simulink model "test_other_torques_sim"  (R2021b)
settings: Solver=ode8  StartTime=0.0  StopTime=1000  FixedStep=0.01  RelTol=1e-3
values from neighbouring files (symbols this model uses):
  alfaG = 0    [test_other_torques_var.m]
  m = [0.1 0.1 0.1]'    [test_other_torques_var.m]
libraries: environment x5, orbit x3, kinematics x3, dynamics x3, my_math_ops x2
settings Model: Creator=Davide  LastModifiedBy=Davide

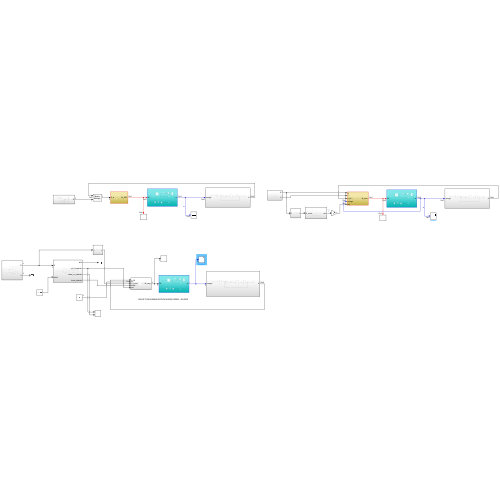
[thumbnail: Simulink's stored preview of the top-level diagram]
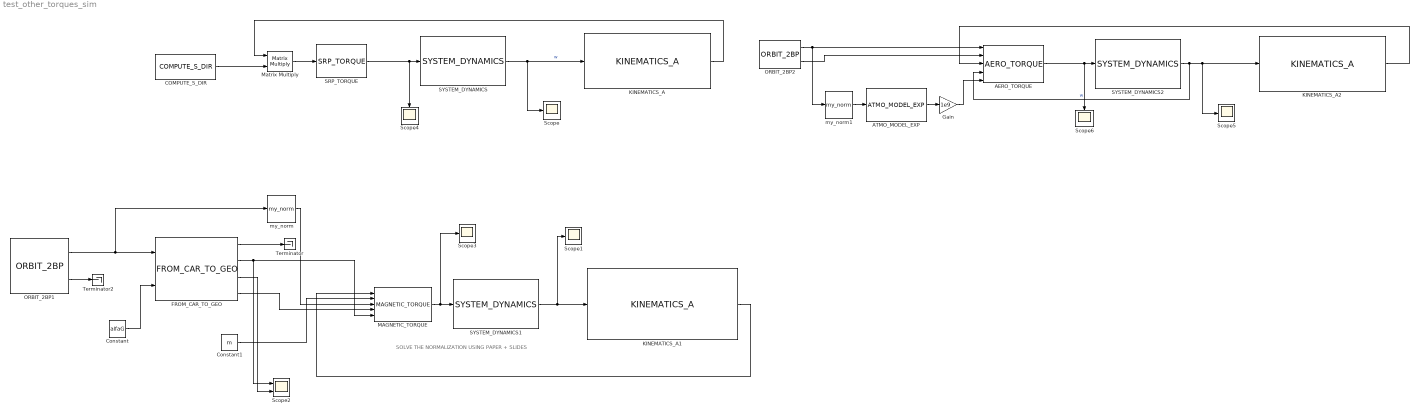
== system test_other_torques_sim ==
  note: SOLVE THE NORMALIZATION USING PAPER + SLIDES
  AERO_TORQUE : environment/AERO_TORQUE  SystemSampleTime=-1  VariantActivationTime=update diagram  Latency=0  AutoFrameSizeCalculation=off
      settings: SourceProductName=Environment
  ATMO_MODEL_EXP : environment/ATMO_MODEL_EXP  SystemSampleTime=-1  VariantActivationTime=update diagram  Latency=0  AutoFrameSizeCalculation=off
      settings: SourceProductName=Environment
  COMPUTE_S_DIR : environment/COMPUTE_S_DIR  SystemSampleTime=-1  VariantActivationTime=update diagram  Latency=0  AutoFrameSizeCalculation=off
      settings: SourceProductName=Environment
  Constant : Constant  Value=alfaG
  Constant1 : Constant  Value=m
  FROM_CAR_TO_GEO : orbit/FROM_CAR_TO_GEO  SystemSampleTime=-1  VariantActivationTime=update diagram  Latency=0  AutoFrameSizeCalculation=off
      settings: SourceProductName=Orbit
  Gain : Gain  Gain=1e9
  KINEMATICS_A : kinematics/KINEMATICS_A  SystemSampleTime=-1  VariantActivationTime=update diagram  Latency=0  AutoFrameSizeCalculation=off
      settings: SourceProductName=Kinematics
  KINEMATICS_A1 : kinematics/KINEMATICS_A  SystemSampleTime=-1  VariantActivationTime=update diagram  Latency=0  AutoFrameSizeCalculation=off
      settings: SourceProductName=Kinematics
  KINEMATICS_A2 : kinematics/KINEMATICS_A  SystemSampleTime=-1  VariantActivationTime=update diagram  Latency=0  AutoFrameSizeCalculation=off
      settings: SourceProductName=Kinematics
  MAGNETIC_TORQUE : environment/MAGNETIC_TORQUE  SystemSampleTime=-1  VariantActivationTime=update diagram  Latency=0  AutoFrameSizeCalculation=off
      settings: SourceProductName=Environment
  Matrix Multiply : Product  Multiplication=Matrix(*)
  ORBIT_2BP1 : orbit/ORBIT_2BP  SystemSampleTime=-1  VariantActivationTime=update diagram  Latency=0  AutoFrameSizeCalculation=off
      settings: SourceProductName=Orbit
  ORBIT_2BP2 : orbit/ORBIT_2BP  SystemSampleTime=-1  VariantActivationTime=update diagram  Latency=0  AutoFrameSizeCalculation=off
      settings: SourceProductName=Orbit
  SRP_TORQUE : environment/SRP_TORQUE  SystemSampleTime=-1  VariantActivationTime=update diagram  Latency=0  AutoFrameSizeCalculation=off
      settings: SourceProductName=Environment
  SYSTEM_DYNAMICS : dynamics/SYSTEM_DYNAMICS  SystemSampleTime=-1  VariantActivationTime=update diagram  Latency=0  AutoFrameSizeCalculation=off
      settings: SourceProductName=Dynamics
  SYSTEM_DYNAMICS1 : dynamics/SYSTEM_DYNAMICS  SystemSampleTime=-1  VariantActivationTime=update diagram  Latency=0  AutoFrameSizeCalculation=off
      settings: SourceProductName=Dynamics
  SYSTEM_DYNAMICS2 : dynamics/SYSTEM_DYNAMICS  SystemSampleTime=-1  VariantActivationTime=update diagram  Latency=0  AutoFrameSizeCalculation=off
      settings: SourceProductName=Dynamics
  Scope{,1,3..6} (6 alike) : Scope
  Scope2 : Scope  NumInputPorts=2
  Terminator : Terminator
  Terminator2 : Terminator
  my_norm : my_math_ops/my_norm  SystemSampleTime=-1  VariantActivationTime=update diagram  Latency=0  AutoFrameSizeCalculation=off
      settings: SourceProductName=My Mathematics Operations
  my_norm1 : my_math_ops/my_norm  SystemSampleTime=-1  VariantActivationTime=update diagram  Latency=0  AutoFrameSizeCalculation=off
      settings: SourceProductName=My Mathematics Operations
  wires:
  SRP_TORQUE/1 -> Scope4/1, SYSTEM_DYNAMICS/1
  SYSTEM_DYNAMICS/1 -> Scope/1, KINEMATICS_A/1  "w"
  KINEMATICS_A1/1 -> MAGNETIC_TORQUE/1
  SYSTEM_DYNAMICS1/1 -> Scope1/1, KINEMATICS_A1/1
  MAGNETIC_TORQUE/1 -> Scope3/1, SYSTEM_DYNAMICS1/1
  ORBIT_2BP1/1 -> my_norm/1, FROM_CAR_TO_GEO/1
  FROM_CAR_TO_GEO/3 -> Scope2/2
  FROM_CAR_TO_GEO/2 -> Scope2/1, MAGNETIC_TORQUE/5
  FROM_CAR_TO_GEO/1 -> Terminator/1
  FROM_CAR_TO_GEO/4 -> MAGNETIC_TORQUE/4
  Constant/1 -> FROM_CAR_TO_GEO/2
  ORBIT_2BP1/2 -> Terminator2/1
  Constant1/1 -> MAGNETIC_TORQUE/2
  my_norm/1 -> MAGNETIC_TORQUE/3
  COMPUTE_S_DIR/1 -> Matrix Multiply/2
  KINEMATICS_A/1 -> Matrix Multiply/1
  Matrix Multiply/1 -> SRP_TORQUE/1
  ORBIT_2BP2/1 -> AERO_TORQUE/1, my_norm1/1
  ORBIT_2BP2/2 -> AERO_TORQUE/2
  KINEMATICS_A2/1 -> AERO_TORQUE/3
  AERO_TORQUE/1 -> Scope6/1, SYSTEM_DYNAMICS2/1
  SYSTEM_DYNAMICS2/1 -> AERO_TORQUE/4, Scope5/1, KINEMATICS_A2/1  "w"
  my_norm1/1 -> ATMO_MODEL_EXP/1
  ATMO_MODEL_EXP/1 -> Gain/1
  Gain/1 -> AERO_TORQUE/5
